simulink model "Demo_Multiple_Quad"  (Simulink 7.7)
settings: Solver=ode4  StartTime=0.0  StopTime=inf  FixedStep=sample_time_Vicon  RelTol=1e-3
InitFcn:
  | sample_time_Vicon = 0.005;
  | sample_time=0.02;
  | DeltaT = sample_time;
  | H0 = 0.35;
  | Kl = 1;
  | Omega_r =1.2; %1.3
  | omega_circle = 36*pi/180;
  | PI = pi;
undefined symbols (not defined in the file or in its folder): DiscIntNeverNeededParam
libraries: simulink x22, dspadpt3 x8
(part 2 of 4)

== system Demo_Multiple_Quad/Quad 6 Planning/Yaw Controller ==
  UAV Bus : Inport
  Bus Selector1 : BusSelector  OutputSignals=Attitude,attitude des,rc
  Gain : Gain  Gain=180/pi
  Heading : simulink/Continuous/PID Controller  SystemSampleTime=-1  Controller=PI  TimeDomain=Discrete-time  SampleTime=sample_time  IntegratorMethod=Trapezoidal  FilterMethod=Trapezoidal  Form=Parallel  P=2  I=1  D=0  N=100  InitialConditionSource=internal  InitialConditionForIntegrator=0  InitialConditionForFilter=0  ExternalReset=rising  LimitOutput=on  UpperSaturationLimit=300*pi/180  LowerSaturationLimit=-300*pi/180  LinearizeAsGain=off  AntiWindupMode=none  Kb=1  TrackingMode=off  Kt=1  PParamMin=[]  PParamMax=[]  IParamMin=[]  IParamMax=[]  DParamMin=[]  DParamMax=[]  NParamMin=[]  NParamMax=[]  KbParamMin=[]  KbParamMax=[]  KtParamMin=[]  KtParamMax=[]  POutMin=[]  POutMax=[]  IOutMin=[]  IOutMax=[]  DOutMin=[]  DOutMax=[]  NOutMin=[]  NOutMax=[]  KbOutMin=[]  KbOutMax=[]  KtOutMin=[]  KtOutMax=[]  IntegratorOutMin=[]  IntegratorOutMax=[]  FilterOutMin=[]  FilterOutMax=[]  SumOutMin=[]  SumOutMax=[]  SumI1OutMin=[]  SumI1OutMax=[]  SumI2OutMin=[]  SumI2OutMax=[]  SumI3OutMin=[]  SumI3OutMax=[]  SumDOutMin=[]  SumDOutMax=[]  SaturationOutMin=[]  SaturationOutMax=[]  IntegratorContinuousStateAttributes=''  IntegratorStateMustResolveToSignalObject=off  IntegratorRTWStateStorageClass=Auto  FilterContinuousStateAttributes=''  FilterStateMustResolveToSignalObject=off  FilterRTWStateStorageClass=Auto
  MATLAB Function : Stateflow chart  TreatAsAtomicUnit=on
  Selector5 : Selector  InputPortWidth=3  IndexOptions=Index vector (dialog)  Indices=[3]  OutputSizes=1
  Selector6 : Selector  InputPortWidth=3  IndexOptions=Index vector (dialog)  Indices=[3]  OutputSizes=1
  Selector7 : Selector  InputPortWidth=8  IndexOptions=Index vector (dialog)  Indices=[5]  OutputSizes=1
  Sum1 : Sum  Inputs=|-+
  Yaw rate des : Outport
  wires:
  Bus Selector1/3 -> Selector7/1  "<rc>"
  Bus Selector1/2 -> Selector6/1  "<attitude des>"
  Selector6/1 -> Sum1/2
  Sum1/1 -> MATLAB Function/1(u)
  MATLAB Function/1(y) -> Heading/1
  UAV Bus/1 -> Bus Selector1/1
  Bus Selector1/1 -> Selector5/1  "<Attitude>"
  Heading/1 -> Gain/1  "desire yaw rate"
  Selector7/1 -> Heading/2  "reset"
  Selector5/1 -> Sum1/1
  Gain/1 -> Yaw rate des/1

== system Demo_Multiple_Quad/Quad 7 Planning/Horizontal Pos controller ==
  UAV Bus : Inport
  Bus Selector : BusSelector  OutputSignals=Position,position des
  Horizontal Position Controller : Subsystem
  Mux : Mux  Inputs=2
  p vs pdes : Scope
      settings: YMin=-1.1  YMax=0.5
  RPY : Outport
  wires:
  UAV Bus/1 -> Horizontal Position Controller/1(UAV Bus), Bus Selector/1
  Horizontal Position Controller/1(RPY) -> RPY/1
  Bus Selector/1 -> Mux/1  "<Position>"
  Bus Selector/2 -> Mux/2  "<position des>"
  Mux/1 -> p vs pdes/1

== system Demo_Multiple_Quad/Quad 7 Planning/Mixer ==
  note: 7x1 vector (usec, XYZRPY)
  RP : Inport
  T : Inport  Port=2
  Yaw rate : Inport  Port=3
  Gain : Gain  Gain=180/pi
  Mux1 : Mux  Inputs=5
  PWM : Constant  Value=0
  "[-1, 1]" : Fcn  Expr=u(1)*2-1
  id : Constant  Value=7
  XYZ RPY : Outport
  wires:
  Mux1/1 -> XYZ RPY/1
  T/1 -> "[-1, 1]"/1
  RP/1 -> Gain/1
  Yaw rate/1 -> Mux1/3
  PWM/1 -> Mux1/4
  id/1 -> Mux1/5
  Gain/1 -> Mux1/2
  "[-1, 1]"/1 -> Mux1/1

== system Demo_Multiple_Quad/Quad 7 Planning/Trajectory Logic ==
  UAV Bus : Inport
  PerchPos : Inport  Port=2
  Bus Selector : BusSelector  OutputSignals=rc,Position,Attitude
  CommandRefSystem : Subsystem
  Mux : Mux  Inputs=2
  Selector1 : Selector  InputPortWidth=3  IndexOptions=Index vector (dialog)  Indices=[3]  OutputSizes=1
  UAV SF1 : Stateflow chart  TreatAsAtomicUnit=on
  PosRef : Outport
  attitude des : Outport  Port=2
  VelRef : Outport  Port=3
  AccRef : Outport  Port=4
  HoverThrottle : Outport  Port=5
  Mode : Outport  Port=6
  wires:
  UAV SF1/1(PosDesired) -> CommandRefSystem/1(PosCom)
  CommandRefSystem/1(position des) -> PosRef/1
  CommandRefSystem/3(velocity des) -> VelRef/1
  Bus Selector/1 -> UAV SF1/1(RC)  "<rc>"
  CommandRefSystem/4(acc des) -> AccRef/1
  UAV SF1/2(HoverThrottle) -> HoverThrottle/1
  PerchPos/1 -> UAV SF1/3(PerchPos)
  UAV SF1/3(Mode) -> Mode/1
  UAV Bus/1 -> Bus Selector/1
  CommandRefSystem/2(attitude des) -> attitude des/1
  Bus Selector/2 -> Mux/1  "<Position>"
  Bus Selector/3 -> Selector1/1  "<Attitude>"
  Selector1/1 -> Mux/2
  Mux/1 -> UAV SF1/2(Pos)

== system Demo_Multiple_Quad/Quad 7 Planning/Vertical Controller ==
  note: Manual Thrust
  UAV bus : Inport
  Hover Throttle : Inport  Port=2
  RP Cmd : Inport  Port=3
  Bus Selector : BusSelector  OutputSignals=Position,position des,rc,velocity,velocity des
  Bus Selector3 : BusSelector  OutputSignals=rc
  Compensation for T from RP cmd : Fcn  Expr=u(1)/(cos(u(2))*cos(u(3)))
  Mux1 : Mux  Inputs=2
  Selector{1,3..5} (4 alike) : Selector  InputPortWidth=3  IndexOptions=Index vector (dialog)  Indices=[3]  OutputSizes=1
  Selector2 : Selector  InputPortWidth=8  IndexOptions=Index vector (dialog)  Indices=[1]  OutputSizes=1
  Selector7 : Selector  InputPortWidth=8  IndexOptions=Index vector (dialog)  Indices=[7]  OutputSizes=1
  Sum : Sum  Inputs=|-+
  Sum1 : Sum  Inputs=|-+
  Verticall Pos Controller : Subsystem
  T : Outport
  wires:
  UAV bus/1 -> Bus Selector/1
  Bus Selector/3 -> Bus Selector3/1, Selector2/1  "<rc>"
  Bus Selector/1 -> Selector4/1  "<Position>"
  Bus Selector/2 -> Selector1/1  "<position des>"
  Sum/1 -> Verticall Pos Controller/1(Pos Error)  "Down error"
  Selector4/1 -> Sum/1
  Selector1/1 -> Sum/2
  Bus Selector3/1 -> Selector7/1  "<rc>"
  Selector7/1 -> Verticall Pos Controller/2(Reset)  "reset"
  Sum1/1 -> Verticall Pos Controller/3(Vel Error)  "Vel_error"
  Selector3/1 -> Sum1/1
  Selector5/1 -> Sum1/2
  Bus Selector/4 -> Selector3/1  "<velocity>"
  Bus Selector/5 -> Selector5/1  "<velocity des>"
  Hover Throttle/1 -> Verticall Pos Controller/4(Hover Throttle)
  RP Cmd/1 -> Mux1/2
  Mux1/1 -> Compensation for T from RP cmd/1
  Verticall Pos Controller/1("T  Commands [0, 1]") -> Mux1/1  "T"
  Compensation for T from RP cmd/1 -> T/1

== system Demo_Multiple_Quad/Quad 7 Planning/Yaw Controller ==
  UAV Bus : Inport
  Bus Selector1 : BusSelector  OutputSignals=Attitude,attitude des,rc
  Gain : Gain  Gain=180/pi
  Heading : simulink/Continuous/PID Controller  SystemSampleTime=-1  Controller=PI  TimeDomain=Discrete-time  SampleTime=sample_time  IntegratorMethod=Trapezoidal  FilterMethod=Trapezoidal  Form=Parallel  P=2  I=1  D=0  N=100  InitialConditionSource=internal  InitialConditionForIntegrator=0  InitialConditionForFilter=0  ExternalReset=rising  LimitOutput=on  UpperSaturationLimit=300*pi/180  LowerSaturationLimit=-300*pi/180  LinearizeAsGain=off  AntiWindupMode=none  Kb=1  TrackingMode=off  Kt=1  PParamMin=[]  PParamMax=[]  IParamMin=[]  IParamMax=[]  DParamMin=[]  DParamMax=[]  NParamMin=[]  NParamMax=[]  KbParamMin=[]  KbParamMax=[]  KtParamMin=[]  KtParamMax=[]  POutMin=[]  POutMax=[]  IOutMin=[]  IOutMax=[]  DOutMin=[]  DOutMax=[]  NOutMin=[]  NOutMax=[]  KbOutMin=[]  KbOutMax=[]  KtOutMin=[]  KtOutMax=[]  IntegratorOutMin=[]  IntegratorOutMax=[]  FilterOutMin=[]  FilterOutMax=[]  SumOutMin=[]  SumOutMax=[]  SumI1OutMin=[]  SumI1OutMax=[]  SumI2OutMin=[]  SumI2OutMax=[]  SumI3OutMin=[]  SumI3OutMax=[]  SumDOutMin=[]  SumDOutMax=[]  SaturationOutMin=[]  SaturationOutMax=[]  IntegratorContinuousStateAttributes=''  IntegratorStateMustResolveToSignalObject=off  IntegratorRTWStateStorageClass=Auto  FilterContinuousStateAttributes=''  FilterStateMustResolveToSignalObject=off  FilterRTWStateStorageClass=Auto
  MATLAB Function : Stateflow chart  TreatAsAtomicUnit=on
  Selector5 : Selector  InputPortWidth=3  IndexOptions=Index vector (dialog)  Indices=[3]  OutputSizes=1
  Selector6 : Selector  InputPortWidth=3  IndexOptions=Index vector (dialog)  Indices=[3]  OutputSizes=1
  Selector7 : Selector  InputPortWidth=8  IndexOptions=Index vector (dialog)  Indices=[5]  OutputSizes=1
  Sum1 : Sum  Inputs=|-+
  Yaw rate des : Outport
  wires:
  Gain/1 -> Yaw rate des/1
  Selector5/1 -> Sum1/1
  Selector7/1 -> Heading/2  "reset"
  Heading/1 -> Gain/1  "desire yaw rate"
  Bus Selector1/1 -> Selector5/1  "<Attitude>"
  UAV Bus/1 -> Bus Selector1/1
  MATLAB Function/1(y) -> Heading/1
  Sum1/1 -> MATLAB Function/1(u)
  Selector6/1 -> Sum1/2
  Bus Selector1/2 -> Selector6/1  "<attitude des>"
  Bus Selector1/3 -> Selector7/1  "<rc>"

== system Demo_Multiple_Quad/Quad 8 Planning /Horizontal Pos controller ==
  UAV Bus : Inport
  Bus Selector : BusSelector  OutputSignals=Position,Attitude,velocity,position des,attitude des,velocity des,rc,Acc des
  Horizontal Position Controller : Subsystem
  RP Cmd : Outport
  wires:
  Horizontal Position Controller/1(RP Cmd) -> RP Cmd/1
  UAV Bus/1 -> Bus Selector/1, Horizontal Position Controller/1(UAV Bus)

== system Demo_Multiple_Quad/Quad 8 Planning /Mixer ==
  note: 7x1 vector (usec, XYZRPY)
  RP : Inport
  T : Inport  Port=2
  Yaw rate : Inport  Port=3
  Gain : Gain  Gain=180/pi
  Mux1 : Mux  Inputs=5
  PWM : Constant  Value=0
  "[-1, 1]" : Fcn  Expr=u(1)*2-1
  id : Constant  Value=8
  XYZ RPY : Outport
  wires:
  id/1 -> Mux1/5
  PWM/1 -> Mux1/4
  Yaw rate/1 -> Mux1/3
  RP/1 -> Gain/1
  T/1 -> "[-1, 1]"/1
  Mux1/1 -> XYZ RPY/1
  Gain/1 -> Mux1/2
  "[-1, 1]"/1 -> Mux1/1

== system Demo_Multiple_Quad/Quad 8 Planning /Trajectory Logic ==
  UAV Bus : Inport
  PerchPos : Inport  Port=2
  Bus Selector : BusSelector  OutputSignals=rc,Position,Attitude
  CommandRefSystem : Subsystem
  Mux : Mux  Inputs=2
  Selector1 : Selector  InputPortWidth=3  IndexOptions=Index vector (dialog)  Indices=[3]  OutputSizes=1
  UAV SF : Stateflow chart  TreatAsAtomicUnit=on
  PosRef : Outport
  attitude des : Outport  Port=2
  VelRef : Outport  Port=3
  AccRef : Outport  Port=4
  HoverThrottle : Outport  Port=5
  Mode : Outport  Port=6
  wires:
  Mux/1 -> UAV SF/2(Pos)
  Selector1/1 -> Mux/2
  Bus Selector/3 -> Selector1/1  "<Attitude>"
  Bus Selector/2 -> Mux/1  "<Position>"
  CommandRefSystem/2(attitude des) -> attitude des/1
  UAV Bus/1 -> Bus Selector/1
  UAV SF/3(Mode) -> Mode/1
  PerchPos/1 -> UAV SF/3(PerchPos)
  UAV SF/2(HoverThrottle) -> HoverThrottle/1
  CommandRefSystem/4(acc des) -> AccRef/1
  Bus Selector/1 -> UAV SF/1(RC)  "<rc>"
  CommandRefSystem/3(velocity des) -> VelRef/1
  CommandRefSystem/1(position des) -> PosRef/1
  UAV SF/1(PosDesired) -> CommandRefSystem/1(PosCom)

== system Demo_Multiple_Quad/Quad 8 Planning /Vertical Controller ==
  note: Manual Thrust
  UAV bus : Inport
  Hover Throttle : Inport  Port=2
  RP Cmd : Inport  Port=3
  Bus Selector : BusSelector  OutputSignals=Position,position des,rc,velocity,velocity des
  Bus Selector3 : BusSelector  OutputSignals=rc
  Compensation for T from RP cmd : Fcn  Expr=u(1)/(cos(u(2))*cos(u(3)))
  Mux1 : Mux  Inputs=2
  Selector{1,3..5} (4 alike) : Selector  InputPortWidth=3  IndexOptions=Index vector (dialog)  Indices=[3]  OutputSizes=1
  Selector2 : Selector  InputPortWidth=8  IndexOptions=Index vector (dialog)  Indices=[1]  OutputSizes=1
  Selector7 : Selector  InputPortWidth=8  IndexOptions=Index vector (dialog)  Indices=[7]  OutputSizes=1
  Sum : Sum  Inputs=|-+
  Sum1 : Sum  Inputs=|-+
  Verticall Pos Controller : Subsystem
  T : Outport
  wires:
  Compensation for T from RP cmd/1 -> T/1
  Mux1/1 -> Compensation for T from RP cmd/1
  RP Cmd/1 -> Mux1/2
  Hover Throttle/1 -> Verticall Pos Controller/4(Hover Throttle)
  Verticall Pos Controller/1("T  Commands [0, 1]") -> Mux1/1  "T"
  Bus Selector/5 -> Selector5/1  "<velocity des>"
  Bus Selector/4 -> Selector3/1  "<velocity>"
  Selector5/1 -> Sum1/2
  Selector3/1 -> Sum1/1
  Sum1/1 -> Verticall Pos Controller/3(Vel Error)  "Vel_error"
  Selector7/1 -> Verticall Pos Controller/2(Reset)  "reset"
  Bus Selector3/1 -> Selector7/1  "<rc>"
  Selector1/1 -> Sum/2
  Selector4/1 -> Sum/1
  Sum/1 -> Verticall Pos Controller/1(Pos Error)  "Down error"
  Bus Selector/2 -> Selector1/1  "<position des>"
  Bus Selector/1 -> Selector4/1  "<Position>"
  Bus Selector/3 -> Selector2/1, Bus Selector3/1  "<rc>"
  UAV bus/1 -> Bus Selector/1

== system Demo_Multiple_Quad/Quad 8 Planning /Yaw Controller ==
  UAV Bus : Inport
  Bus Selector1 : BusSelector  OutputSignals=Attitude,attitude des,rc
  Gain : Gain  Gain=180/pi
  Heading : simulink/Continuous/PID Controller  SystemSampleTime=-1  Controller=PI  TimeDomain=Discrete-time  SampleTime=sample_time  IntegratorMethod=Trapezoidal  FilterMethod=Trapezoidal  Form=Parallel  P=2  I=1  D=0  N=100  InitialConditionSource=internal  InitialConditionForIntegrator=0  InitialConditionForFilter=0  ExternalReset=rising  LimitOutput=on  UpperSaturationLimit=300*pi/180  LowerSaturationLimit=-300*pi/180  LinearizeAsGain=off  AntiWindupMode=none  Kb=1  TrackingMode=off  Kt=1  PParamMin=[]  PParamMax=[]  IParamMin=[]  IParamMax=[]  DParamMin=[]  DParamMax=[]  NParamMin=[]  NParamMax=[]  KbParamMin=[]  KbParamMax=[]  KtParamMin=[]  KtParamMax=[]  POutMin=[]  POutMax=[]  IOutMin=[]  IOutMax=[]  DOutMin=[]  DOutMax=[]  NOutMin=[]  NOutMax=[]  KbOutMin=[]  KbOutMax=[]  KtOutMin=[]  KtOutMax=[]  IntegratorOutMin=[]  IntegratorOutMax=[]  FilterOutMin=[]  FilterOutMax=[]  SumOutMin=[]  SumOutMax=[]  SumI1OutMin=[]  SumI1OutMax=[]  SumI2OutMin=[]  SumI2OutMax=[]  SumI3OutMin=[]  SumI3OutMax=[]  SumDOutMin=[]  SumDOutMax=[]  SaturationOutMin=[]  SaturationOutMax=[]  IntegratorContinuousStateAttributes=''  IntegratorStateMustResolveToSignalObject=off  IntegratorRTWStateStorageClass=Auto  FilterContinuousStateAttributes=''  FilterStateMustResolveToSignalObject=off  FilterRTWStateStorageClass=Auto
  MATLAB Function : Stateflow chart  TreatAsAtomicUnit=on
  Selector5 : Selector  InputPortWidth=3  IndexOptions=Index vector (dialog)  Indices=[3]  OutputSizes=1
  Selector6 : Selector  InputPortWidth=3  IndexOptions=Index vector (dialog)  Indices=[3]  OutputSizes=1
  Selector7 : Selector  InputPortWidth=8  IndexOptions=Index vector (dialog)  Indices=[5]  OutputSizes=1
  Sum1 : Sum  Inputs=|-+
  Yaw rate des : Outport
  wires:
  Bus Selector1/3 -> Selector7/1  "<rc>"
  Bus Selector1/2 -> Selector6/1  "<attitude des>"
  Selector6/1 -> Sum1/2
  Sum1/1 -> MATLAB Function/1(u)
  MATLAB Function/1(y) -> Heading/1
  UAV Bus/1 -> Bus Selector1/1
  Bus Selector1/1 -> Selector5/1  "<Attitude>"
  Heading/1 -> Gain/1  "desire yaw rate"
  Selector7/1 -> Heading/2  "reset"
  Selector5/1 -> Sum1/1
  Gain/1 -> Yaw rate des/1

== system Demo_Multiple_Quad/Vicon_Data/Filter1 ==
  In1 : Inport
  Gain : Gain  Gain=15
  Integrator : Integrator
  Kalman Filter : dspadpt3/Kalman Filter  SystemSampleTime=-1  num_targets=1  sourceEnable=Always  isReset=on  X=zeros([9, 1])  P=zeros(9)  A=[1 sample_time_Vicon sample_time_Vicon*sample_time_Vicon/2 zeros(1,6);0 1 sample_time_Vicon zeros(1,6);0 0 1 zeros(1,6);0 0 0 1 sample_time_Vicon sample_time_Vicon*sample_time_Vicon/2 0 0 0;zeros(1,4) 1 sample_time_Vicon zeros(1,3);zeros(1,5) 1 zeros(1,3);zeros(1,6) 1 sample_time_Vicon sample_time_Vicon*sample_time_Vicon/2;zeros(1,7) 1 sample_time_Vicon;zeros(1,8) 1]  sourceMeasure=Specify via Dialog  H=[1 zeros(1,8); zeros(1,3) 1 zeros(1,5);zeros(1,6) 1 0 0]  Q=diag([0 0.001 0.001 0 0.001 0.001 0 0.001 0.001])  R=0.001*eye(3)  isOutputEstMeasure=on  isOutputEstState=on  isOutputEstError=off  isOutputPrdMeasure=off  isOutputPrdState=off  isOutputPrdError=off
  Selector5 : Selector  InputPortWidth=9  IndexOptions=Index vector (dialog)  Indices=[2 5 8]  OutputSizes=1
  Selector6 : Selector  InputPortWidth=9  IndexOptions=Index vector (dialog)  Indices=[3 6 9]  OutputSizes=1
  Sum : Sum  Inputs=|+-
  Pos : Outport
  Vel : Outport  Port=2
  Acc : Outport  Port=3
  wires:
  Selector5/1 -> Vel/1
  Sum/1 -> Gain/1
  Gain/1 -> Integrator/1
  Integrator/1 -> Pos/1, Sum/2
  In1/1 -> Kalman Filter/1, Sum/1
  Kalman Filter/2 -> Selector5/1, Selector6/1
  Selector6/1 -> Acc/1

== system Demo_Multiple_Quad/Vicon_Data/Filter2 ==
  In1 : Inport
  Gain : Gain  Gain=15
  Integrator : Integrator
  Kalman Filter : dspadpt3/Kalman Filter  SystemSampleTime=-1  num_targets=1  sourceEnable=Always  isReset=on  X=zeros([9, 1])  P=zeros(9)  A=[1 sample_time_Vicon sample_time_Vicon*sample_time_Vicon/2 zeros(1,6);0 1 sample_time_Vicon zeros(1,6);0 0 1 zeros(1,6);0 0 0 1 sample_time_Vicon sample_time_Vicon*sample_time_Vicon/2 0 0 0;zeros(1,4) 1 sample_time_Vicon zeros(1,3);zeros(1,5) 1 zeros(1,3);zeros(1,6) 1 sample_time_Vicon sample_time_Vicon*sample_time_Vicon/2;zeros(1,7) 1 sample_time_Vicon;zeros(1,8) 1]  sourceMeasure=Specify via Dialog  H=[1 zeros(1,8); zeros(1,3) 1 zeros(1,5);zeros(1,6) 1 0 0]  Q=diag([0 0.001 0.001 0 0.001 0.001 0 0.001 0.001])  R=0.001*eye(3)  isOutputEstMeasure=on  isOutputEstState=on  isOutputEstError=off  isOutputPrdMeasure=off  isOutputPrdState=off  isOutputPrdError=off
  Selector5 : Selector  InputPortWidth=9  IndexOptions=Index vector (dialog)  Indices=[2 5 8]  OutputSizes=1
  Selector6 : Selector  InputPortWidth=9  IndexOptions=Index vector (dialog)  Indices=[3 6 9]  OutputSizes=1
  Sum : Sum  Inputs=|+-
  Pos : Outport
  Vel : Outport  Port=2
  Acc : Outport  Port=3
  wires:
  Selector6/1 -> Acc/1
  Kalman Filter/2 -> Selector6/1, Selector5/1
  In1/1 -> Sum/1, Kalman Filter/1
  Integrator/1 -> Sum/2, Pos/1
  Gain/1 -> Integrator/1
  Sum/1 -> Gain/1
  Selector5/1 -> Vel/1

== system Demo_Multiple_Quad/Vicon_Data/Filter3 ==
  In1 : Inport
  Gain : Gain  Gain=15
  Integrator : Integrator
  Kalman Filter : dspadpt3/Kalman Filter  SystemSampleTime=-1  num_targets=1  sourceEnable=Always  isReset=on  X=zeros([9, 1])  P=zeros(9)  A=[1 sample_time_Vicon sample_time_Vicon*sample_time_Vicon/2 zeros(1,6);0 1 sample_time_Vicon zeros(1,6);0 0 1 zeros(1,6);0 0 0 1 sample_time_Vicon sample_time_Vicon*sample_time_Vicon/2 0 0 0;zeros(1,4) 1 sample_time_Vicon zeros(1,3);zeros(1,5) 1 zeros(1,3);zeros(1,6) 1 sample_time_Vicon sample_time_Vicon*sample_time_Vicon/2;zeros(1,7) 1 sample_time_Vicon;zeros(1,8) 1]  sourceMeasure=Specify via Dialog  H=[1 zeros(1,8); zeros(1,3) 1 zeros(1,5);zeros(1,6) 1 0 0]  Q=diag([0 0.001 0.001 0 0.001 0.001 0 0.001 0.001])  R=0.001*eye(3)  isOutputEstMeasure=on  isOutputEstState=on  isOutputEstError=off  isOutputPrdMeasure=off  isOutputPrdState=off  isOutputPrdError=off
  Selector5 : Selector  InputPortWidth=9  IndexOptions=Index vector (dialog)  Indices=[2 5 8]  OutputSizes=1
  Selector6 : Selector  InputPortWidth=9  IndexOptions=Index vector (dialog)  Indices=[3 6 9]  OutputSizes=1
  Sum : Sum  Inputs=|+-
  Pos : Outport
  Vel : Outport  Port=2
  Acc : Outport  Port=3
  wires:
  Selector5/1 -> Vel/1
  Sum/1 -> Gain/1
  Gain/1 -> Integrator/1
  Integrator/1 -> Pos/1, Sum/2
  In1/1 -> Kalman Filter/1, Sum/1
  Kalman Filter/2 -> Selector5/1, Selector6/1
  Selector6/1 -> Acc/1

== system Demo_Multiple_Quad/Vicon_Data/Filter4 ==
  In1 : Inport
  Gain : Gain  Gain=15
  Integrator : Integrator
  Kalman Filter : dspadpt3/Kalman Filter  SystemSampleTime=-1  num_targets=1  sourceEnable=Always  isReset=on  X=zeros([9, 1])  P=zeros(9)  A=[1 sample_time_Vicon sample_time_Vicon*sample_time_Vicon/2 zeros(1,6);0 1 sample_time_Vicon zeros(1,6);0 0 1 zeros(1,6);0 0 0 1 sample_time_Vicon sample_time_Vicon*sample_time_Vicon/2 0 0 0;zeros(1,4) 1 sample_time_Vicon zeros(1,3);zeros(1,5) 1 zeros(1,3);zeros(1,6) 1 sample_time_Vicon sample_time_Vicon*sample_time_Vicon/2;zeros(1,7) 1 sample_time_Vicon;zeros(1,8) 1]  sourceMeasure=Specify via Dialog  H=[1 zeros(1,8); zeros(1,3) 1 zeros(1,5);zeros(1,6) 1 0 0]  Q=diag([0 0.001 0.001 0 0.001 0.001 0 0.001 0.001])  R=0.001*eye(3)  isOutputEstMeasure=on  isOutputEstState=on  isOutputEstError=off  isOutputPrdMeasure=off  isOutputPrdState=off  isOutputPrdError=off
  Selector5 : Selector  InputPortWidth=9  IndexOptions=Index vector (dialog)  Indices=[2 5 8]  OutputSizes=1
  Selector6 : Selector  InputPortWidth=9  IndexOptions=Index vector (dialog)  Indices=[3 6 9]  OutputSizes=1
  Sum : Sum  Inputs=|+-
  Pos : Outport
  Vel : Outport  Port=2
  Acc : Outport  Port=3
  wires:
  Selector6/1 -> Acc/1
  Kalman Filter/2 -> Selector6/1, Selector5/1
  In1/1 -> Sum/1, Kalman Filter/1
  Integrator/1 -> Sum/2, Pos/1
  Gain/1 -> Integrator/1
  Sum/1 -> Gain/1
  Selector5/1 -> Vel/1

== system Demo_Multiple_Quad/Vicon_Data/Filter5 ==
  In1 : Inport
  Gain : Gain  Gain=15
  Integrator : Integrator
  Kalman Filter : dspadpt3/Kalman Filter  SystemSampleTime=-1  num_targets=1  sourceEnable=Always  isReset=on  X=zeros([9, 1])  P=zeros(9)  A=[1 sample_time_Vicon sample_time_Vicon*sample_time_Vicon/2 zeros(1,6);0 1 sample_time_Vicon zeros(1,6);0 0 1 zeros(1,6);0 0 0 1 sample_time_Vicon sample_time_Vicon*sample_time_Vicon/2 0 0 0;zeros(1,4) 1 sample_time_Vicon zeros(1,3);zeros(1,5) 1 zeros(1,3);zeros(1,6) 1 sample_time_Vicon sample_time_Vicon*sample_time_Vicon/2;zeros(1,7) 1 sample_time_Vicon;zeros(1,8) 1]  sourceMeasure=Specify via Dialog  H=[1 zeros(1,8); zeros(1,3) 1 zeros(1,5);zeros(1,6) 1 0 0]  Q=diag([0 0.001 0.001 0 0.001 0.001 0 0.001 0.001])  R=0.001*eye(3)  isOutputEstMeasure=on  isOutputEstState=on  isOutputEstError=off  isOutputPrdMeasure=off  isOutputPrdState=off  isOutputPrdError=off
  Selector5 : Selector  InputPortWidth=9  IndexOptions=Index vector (dialog)  Indices=[2 5 8]  OutputSizes=1
  Selector6 : Selector  InputPortWidth=9  IndexOptions=Index vector (dialog)  Indices=[3 6 9]  OutputSizes=1
  Sum : Sum  Inputs=|+-
  Pos : Outport
  Vel : Outport  Port=2
  Acc : Outport  Port=3
  wires:
  Selector5/1 -> Vel/1
  Sum/1 -> Gain/1
  Gain/1 -> Integrator/1
  Integrator/1 -> Pos/1, Sum/2
  In1/1 -> Kalman Filter/1, Sum/1
  Kalman Filter/2 -> Selector5/1, Selector6/1
  Selector6/1 -> Acc/1

== system Demo_Multiple_Quad/Vicon_Data/Filter6 ==
  In1 : Inport
  Gain : Gain  Gain=15
  Integrator : Integrator
  Kalman Filter : dspadpt3/Kalman Filter  SystemSampleTime=-1  num_targets=1  sourceEnable=Always  isReset=on  X=zeros([9, 1])  P=zeros(9)  A=[1 sample_time_Vicon sample_time_Vicon*sample_time_Vicon/2 zeros(1,6);0 1 sample_time_Vicon zeros(1,6);0 0 1 zeros(1,6);0 0 0 1 sample_time_Vicon sample_time_Vicon*sample_time_Vicon/2 0 0 0;zeros(1,4) 1 sample_time_Vicon zeros(1,3);zeros(1,5) 1 zeros(1,3);zeros(1,6) 1 sample_time_Vicon sample_time_Vicon*sample_time_Vicon/2;zeros(1,7) 1 sample_time_Vicon;zeros(1,8) 1]  sourceMeasure=Specify via Dialog  H=[1 zeros(1,8); zeros(1,3) 1 zeros(1,5);zeros(1,6) 1 0 0]  Q=diag([0 0.001 0.001 0 0.001 0.001 0 0.001 0.001])  R=0.001*eye(3)  isOutputEstMeasure=on  isOutputEstState=on  isOutputEstError=off  isOutputPrdMeasure=off  isOutputPrdState=off  isOutputPrdError=off
  Selector5 : Selector  InputPortWidth=9  IndexOptions=Index vector (dialog)  Indices=[2 5 8]  OutputSizes=1
  Selector6 : Selector  InputPortWidth=9  IndexOptions=Index vector (dialog)  Indices=[3 6 9]  OutputSizes=1
  Sum : Sum  Inputs=|+-
  Pos : Outport
  Vel : Outport  Port=2
  Acc : Outport  Port=3
  wires:
  Selector6/1 -> Acc/1
  Kalman Filter/2 -> Selector6/1, Selector5/1
  In1/1 -> Sum/1, Kalman Filter/1
  Integrator/1 -> Sum/2, Pos/1
  Gain/1 -> Integrator/1
  Sum/1 -> Gain/1
  Selector5/1 -> Vel/1

== system Demo_Multiple_Quad/Vicon_Data/Filter7 ==
  In1 : Inport
  Gain : Gain  Gain=15
  Integrator : Integrator
  Kalman Filter : dspadpt3/Kalman Filter  SystemSampleTime=-1  num_targets=1  sourceEnable=Always  isReset=on  X=zeros([9, 1])  P=zeros(9)  A=[1 sample_time_Vicon sample_time_Vicon*sample_time_Vicon/2 zeros(1,6);0 1 sample_time_Vicon zeros(1,6);0 0 1 zeros(1,6);0 0 0 1 sample_time_Vicon sample_time_Vicon*sample_time_Vicon/2 0 0 0;zeros(1,4) 1 sample_time_Vicon zeros(1,3);zeros(1,5) 1 zeros(1,3);zeros(1,6) 1 sample_time_Vicon sample_time_Vicon*sample_time_Vicon/2;zeros(1,7) 1 sample_time_Vicon;zeros(1,8) 1]  sourceMeasure=Specify via Dialog  H=[1 zeros(1,8); zeros(1,3) 1 zeros(1,5);zeros(1,6) 1 0 0]  Q=diag([0 0.001 0.001 0 0.001 0.001 0 0.001 0.001])  R=0.001*eye(3)  isOutputEstMeasure=on  isOutputEstState=on  isOutputEstError=off  isOutputPrdMeasure=off  isOutputPrdState=off  isOutputPrdError=off
  Selector5 : Selector  InputPortWidth=9  IndexOptions=Index vector (dialog)  Indices=[2 5 8]  OutputSizes=1
  Selector6 : Selector  InputPortWidth=9  IndexOptions=Index vector (dialog)  Indices=[3 6 9]  OutputSizes=1
  Sum : Sum  Inputs=|+-
  Pos : Outport
  Vel : Outport  Port=2
  Acc : Outport  Port=3
  wires:
  Selector6/1 -> Acc/1
  Kalman Filter/2 -> Selector6/1, Selector5/1
  In1/1 -> Sum/1, Kalman Filter/1
  Integrator/1 -> Sum/2, Pos/1
  Gain/1 -> Integrator/1
  Sum/1 -> Gain/1
  Selector5/1 -> Vel/1

== system Demo_Multiple_Quad/Vicon_Data/Filter8 ==
  In1 : Inport
  Gain : Gain  Gain=15
  Integrator : Integrator
  Kalman Filter : dspadpt3/Kalman Filter  SystemSampleTime=-1  num_targets=1  sourceEnable=Always  isReset=on  X=zeros([9, 1])  P=zeros(9)  A=[1 sample_time_Vicon sample_time_Vicon*sample_time_Vicon/2 zeros(1,6);0 1 sample_time_Vicon zeros(1,6);0 0 1 zeros(1,6);0 0 0 1 sample_time_Vicon sample_time_Vicon*sample_time_Vicon/2 0 0 0;zeros(1,4) 1 sample_time_Vicon zeros(1,3);zeros(1,5) 1 zeros(1,3);zeros(1,6) 1 sample_time_Vicon sample_time_Vicon*sample_time_Vicon/2;zeros(1,7) 1 sample_time_Vicon;zeros(1,8) 1]  sourceMeasure=Specify via Dialog  H=[1 zeros(1,8); zeros(1,3) 1 zeros(1,5);zeros(1,6) 1 0 0]  Q=diag([0 0.001 0.001 0 0.001 0.001 0 0.001 0.001])  R=0.001*eye(3)  isOutputEstMeasure=on  isOutputEstState=on  isOutputEstError=off  isOutputPrdMeasure=off  isOutputPrdState=off  isOutputPrdError=off
  Selector5 : Selector  InputPortWidth=9  IndexOptions=Index vector (dialog)  Indices=[2 5 8]  OutputSizes=1
  Selector6 : Selector  InputPortWidth=9  IndexOptions=Index vector (dialog)  Indices=[3 6 9]  OutputSizes=1
  Sum : Sum  Inputs=|+-
  Pos : Outport
  Vel : Outport  Port=2
  Acc : Outport  Port=3
  wires:
  Selector5/1 -> Vel/1
  Sum/1 -> Gain/1
  Gain/1 -> Integrator/1
  Integrator/1 -> Pos/1, Sum/2
  In1/1 -> Kalman Filter/1, Sum/1
  Kalman Filter/2 -> Selector5/1, Selector6/1
  Selector6/1 -> Acc/1

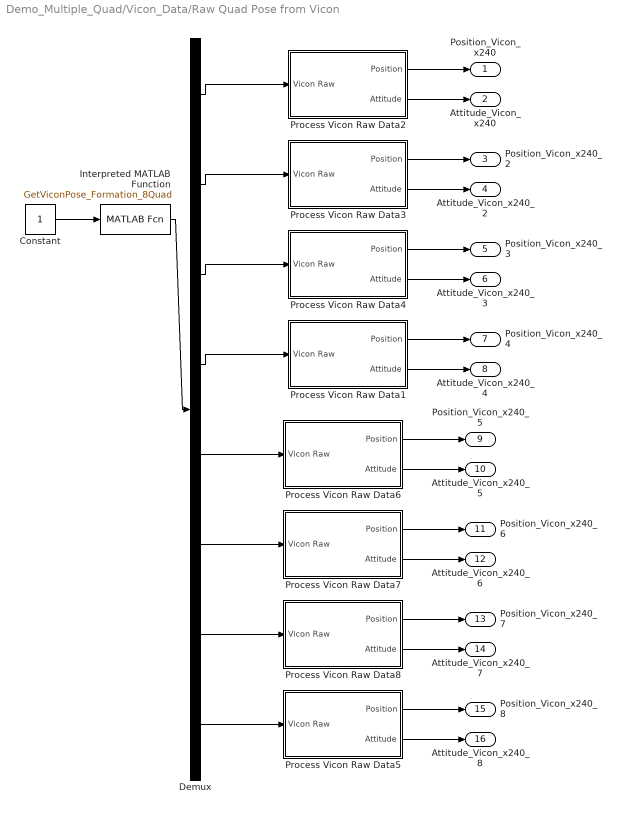
== system Demo_Multiple_Quad/Vicon_Data/Raw Quad Pose from Vicon ==
  Constant : Constant
  Demux : Demux  Outputs=8
  Interpreted MATLAB Function : MATLABFcn  MATLABFcn=GetViconPose_Formation_8Quad
  Process Vicon Raw Data1 : Subsystem
  Process Vicon Raw Data2 : Subsystem
  Process Vicon Raw Data3 : Subsystem
  Process Vicon Raw Data4 : Subsystem
  Process Vicon Raw Data5 : Subsystem
  Process Vicon Raw Data6 : Subsystem
  Process Vicon Raw Data7 : Subsystem
  Process Vicon Raw Data8 : Subsystem
  Position_Vicon_x240 : Outport
  Attitude_Vicon_x240 : Outport  Port=2
  Position_Vicon_x240_2 : Outport  Port=3
  Attitude_Vicon_x240_2 : Outport  Port=4
  Position_Vicon_x240_3 : Outport  Port=5
  Attitude_Vicon_x240_3 : Outport  Port=6
  Position_Vicon_x240_4 : Outport  Port=7
  Attitude_Vicon_x240_4 : Outport  Port=8
  Position_Vicon_x240_5 : Outport  Port=9
  Attitude_Vicon_x240_5 : Outport  Port=10
  Position_Vicon_x240_6 : Outport  Port=11
  Attitude_Vicon_x240_6 : Outport  Port=12
  Position_Vicon_x240_7 : Outport  Port=13
  Attitude_Vicon_x240_7 : Outport  Port=14
  Position_Vicon_x240_8 : Outport  Port=15
  Attitude_Vicon_x240_8 : Outport  Port=16
  wires:
  Process Vicon Raw Data2/2(Attitude) -> Attitude_Vicon_x240/1
  Process Vicon Raw Data2/1(Position) -> Position_Vicon_x240/1
  Constant/1 -> Interpreted MATLAB Function/1
  Interpreted MATLAB Function/1 -> Demux/1
  Process Vicon Raw Data3/2(Attitude) -> Attitude_Vicon_x240_2/1
  Process Vicon Raw Data3/1(Position) -> Position_Vicon_x240_2/1
  Process Vicon Raw Data4/2(Attitude) -> Attitude_Vicon_x240_3/1
  Process Vicon Raw Data4/1(Position) -> Position_Vicon_x240_3/1
  Demux/1 -> Process Vicon Raw Data2/1(Vicon Raw)
  Demux/2 -> Process Vicon Raw Data3/1(Vicon Raw)
  Demux/3 -> Process Vicon Raw Data4/1(Vicon Raw)
  Process Vicon Raw Data1/2(Attitude) -> Attitude_Vicon_x240_4/1
  Process Vicon Raw Data1/1(Position) -> Position_Vicon_x240_4/1
  Demux/4 -> Process Vicon Raw Data1/1(Vicon Raw)
  Process Vicon Raw Data6/2(Attitude) -> Attitude_Vicon_x240_5/1
  Process Vicon Raw Data6/1(Position) -> Position_Vicon_x240_5/1
  Process Vicon Raw Data7/2(Attitude) -> Attitude_Vicon_x240_6/1
  Process Vicon Raw Data7/1(Position) -> Position_Vicon_x240_6/1
  Process Vicon Raw Data8/2(Attitude) -> Attitude_Vicon_x240_7/1
  Process Vicon Raw Data8/1(Position) -> Position_Vicon_x240_7/1
  Demux/5 -> Process Vicon Raw Data6/1(Vicon Raw)
  Demux/6 -> Process Vicon Raw Data7/1(Vicon Raw)
  Demux/7 -> Process Vicon Raw Data8/1(Vicon Raw)
  Process Vicon Raw Data5/2(Attitude) -> Attitude_Vicon_x240_8/1
  Process Vicon Raw Data5/1(Position) -> Position_Vicon_x240_8/1
  Demux/8 -> Process Vicon Raw Data5/1(Vicon Raw)

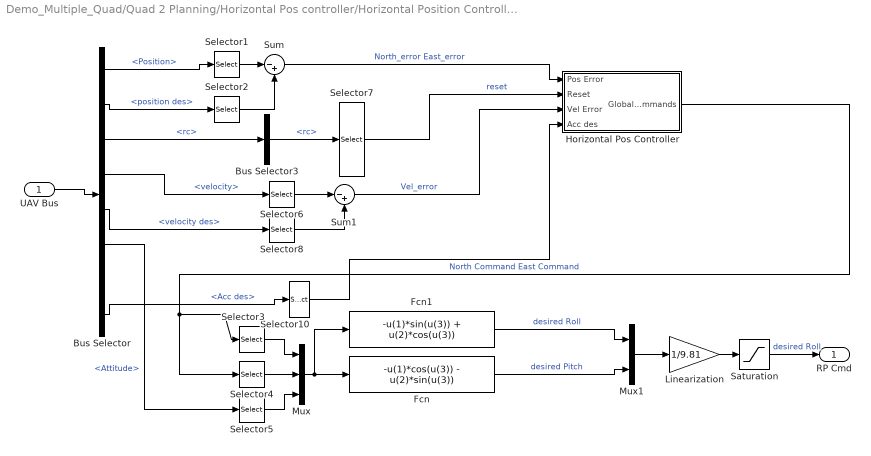
== system Demo_Multiple_Quad/Quad 2 Planning/Horizontal Pos controller/Horizontal Position Controller ==
  UAV Bus : Inport
  Bus Selector : BusSelector  OutputSignals=Position,position des,rc,velocity,velocity des,Attitude,Acceleration,Acc des
  Bus Selector3 : BusSelector  OutputSignals=rc
  Fcn : Fcn  Expr=-u(1)*cos(u(3)) - u(2)*sin(u(3))
  Fcn1 : Fcn  Expr=-u(1)*sin(u(3)) + u(2)*cos(u(3))
  Horizontal Pos Controller : Subsystem
  Linearization : Gain  Gain=1/9.81  OutDataTypeStr=double
  Mux : Mux  Inputs=3
  Mux1 : Mux  Inputs=2
  Saturation : Saturate  UpperLimit=60*pi/180  LowerLimit=-60*pi/180
  Selector{1..2,6,8} (4 alike) : Selector  InputPortWidth=3  IndexOptions=Index vector (dialog)  Indices=[1 2]  OutputSizes=1
  Selector10 : Selector  InputPortWidth=4  IndexOptions=Index vector (dialog)  Indices=[1 2]  OutputSizes=1
  Selector3 : Selector  InputPortWidth=2  IndexOptions=Index vector (dialog)  Indices=[1]  OutputSizes=1
  Selector4 : Selector  InputPortWidth=2  IndexOptions=Index vector (dialog)  Indices=[2]  OutputSizes=1
  Selector5 : Selector  InputPortWidth=3  IndexOptions=Index vector (dialog)  Indices=[3]  OutputSizes=1
  Selector7 : Selector  InputPortWidth=8  IndexOptions=Index vector (dialog)  Indices=[7]  OutputSizes=1
  Sum : Sum  Inputs=|-+
  Sum1 : Sum  Inputs=|-+
  RP Cmd : Outport
  wires:
  Sum/1 -> Horizontal Pos Controller/1(Pos Error)  "North_error East_error"
  Bus Selector/1 -> Selector1/1  "<Position>"
  Bus Selector/2 -> Selector2/1  "<position des>"
  Selector1/1 -> Sum/1
  Selector2/1 -> Sum/2
  UAV Bus/1 -> Bus Selector/1
  Horizontal Pos Controller/1(Global Commands) -> Selector3/1, Selector4/1  "North Command East Command"
  Bus Selector/6 -> Selector5/1  "<Attitude>"
  Selector3/1 -> Mux/1
  Selector4/1 -> Mux/2
  Selector5/1 -> Mux/3
  Mux/1 -> Fcn/1, Fcn1/1
  Fcn1/1 -> Mux1/1  "desired Roll"
  Fcn/1 -> Mux1/2  "desired Pitch"
  Mux1/1 -> Linearization/1
  Bus Selector3/1 -> Selector7/1  "<rc>"
  Selector7/1 -> Horizontal Pos Controller/2(Reset)  "reset"
  Sum1/1 -> Horizontal Pos Controller/3(Vel Error)  "Vel_error"
  Selector6/1 -> Sum1/1
  Selector8/1 -> Sum1/2
  Bus Selector/3 -> Bus Selector3/1  "<rc>"
  Bus Selector/4 -> Selector6/1  "<velocity>"
  Bus Selector/5 -> Selector8/1  "<velocity des>"
  Bus Selector/8 -> Selector10/1  "<Acc des>"
  Selector10/1 -> Horizontal Pos Controller/4(Acc des)
  Linearization/1 -> Saturation/1
  Saturation/1 -> RP Cmd/1  "desired Roll"

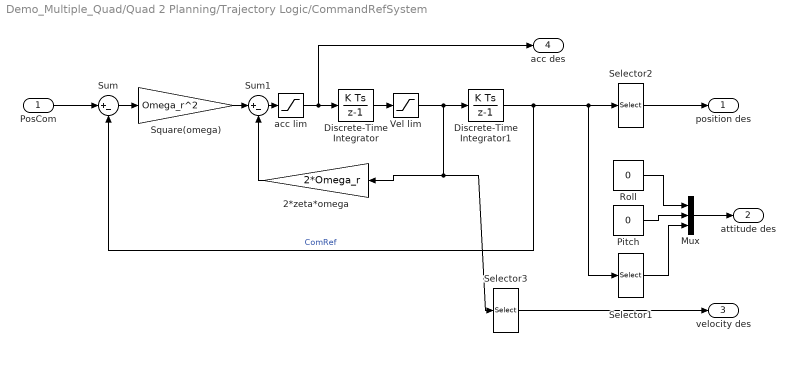
== system Demo_Multiple_Quad/Quad 2 Planning/Trajectory Logic/CommandRefSystem ==
  PosCom : Inport
  2*zeta*omega : Gain  Gain=2*Omega_r
  Discrete-Time Integrator : DiscreteIntegrator  SampleTime=0.02  ICPrevOutput=DiscIntNeverNeededParam  ICPrevScaledInput=DiscIntNeverNeededParam
  Discrete-Time Integrator1 : DiscreteIntegrator  SampleTime=0.02  ICPrevOutput=DiscIntNeverNeededParam  ICPrevScaledInput=DiscIntNeverNeededParam
  Mux : Mux  Inputs=3
  Pitch : Constant  Value=0  SampleTime=0.02
  Roll : Constant  Value=0  SampleTime=0.02
  Selector1 : Selector  InputPortWidth=4  IndexOptions=Index vector (dialog)  Indices=[4]  OutputSizes=1
  Selector2 : Selector  InputPortWidth=4  IndexOptions=Index vector (dialog)  Indices=[1 2 3]  OutputSizes=1
  Selector3 : Selector  InputPortWidth=4  IndexOptions=Index vector (dialog)  Indices=[1 2 3]  OutputSizes=1
  Square(omega) : Gain  Gain=Omega_r^2
  Sum : Sum  Inputs=|+-
  Sum1 : Sum  Inputs=|+-
  Vel lim : Saturate  UpperLimit=3  LowerLimit=-3
  acc lim : Saturate  UpperLimit=4  LowerLimit=-4
  position des : Outport
  attitude des : Outport  Port=2
  velocity des : Outport  Port=3
  acc des : Outport  Port=4
  wires:
  Discrete-Time Integrator1/1 -> Sum/2, Selector2/1, Selector1/1  "ComRef"
  PosCom/1 -> Sum/1
  Sum/1 -> Square(omega)/1
  Square(omega)/1 -> Sum1/1
  Discrete-Time Integrator/1 -> Vel lim/1
  Sum1/1 -> acc lim/1
  2*zeta*omega/1 -> Sum1/2
  Selector2/1 -> position des/1
  Roll/1 -> Mux/1
  Pitch/1 -> Mux/2
  Selector1/1 -> Mux/3
  Mux/1 -> attitude des/1
  Selector3/1 -> velocity des/1
  acc lim/1 -> acc des/1, Discrete-Time Integrator/1
  Vel lim/1 -> 2*zeta*omega/1, Selector3/1, Discrete-Time Integrator1/1

== system Demo_Multiple_Quad/Quad 2 Planning/Vertical Controller/Verticall Pos Controller ==
  note: Set 1:
      | without KF
  note: 0.25
      | 0.1
      | 0.15
  note: Set 1:
      | with KF
  note: 0.15
      | 0.08
      | 0.15
  Pos Error : Inport
  Reset : Inport  Port=2
  Vel Error : Inport  Port=3
  Hover Throttle : Inport  Port=4
  D Gain : Gain  Gain=0.1  OutDataTypeStr=double
  Integral Gain : Gain  DisableCoverage=on  Gain=0.05  ParamDataTypeStr=double  OutDataTypeStr=double
  Integrator : DiscreteIntegrator  DisableCoverage=on  IntegratorMethod=Integration: Trapezoidal  ExternalReset=rising  InitialConditionMode=State only (most efficient)  SampleTime=-1  OutDataTypeStr=double  LimitOutput=on  UpperSaturationLimit=0.3  LowerSaturationLimit=-0.3  ICPrevOutput=DiscIntNeverNeededParam  ICPrevScaledInput=DiscIntNeverNeededParam
  Proportional Gain : Gain  DisableCoverage=on  Gain=0.1  ParamDataTypeStr=double  OutDataTypeStr=double
  Sum1 : Sum  DisableCoverage=on  Inputs=---|  AccumDataTypeStr=double  OutDataTypeStr=double  SampleTime=0.02
  Sum2 : Sum  DisableCoverage=on  Inputs=++|  AccumDataTypeStr=double  OutDataTypeStr=double  SampleTime=0.02
  "T  Commands [0, 1]" : Outport
  wires:
  Integral Gain/1 -> Integrator/1
  Integrator/1 -> Sum1/2
  Proportional Gain/1 -> Sum1/1
  Pos Error/1 -> Proportional Gain/1, Integral Gain/1
  Reset/1 -> Integrator/2
  Vel Error/1 -> D Gain/1
  D Gain/1 -> Sum1/3
  Sum1/1 -> Sum2/1
  Hover Throttle/1 -> Sum2/2
  Sum2/1 -> "T  Commands [0, 1]"/1

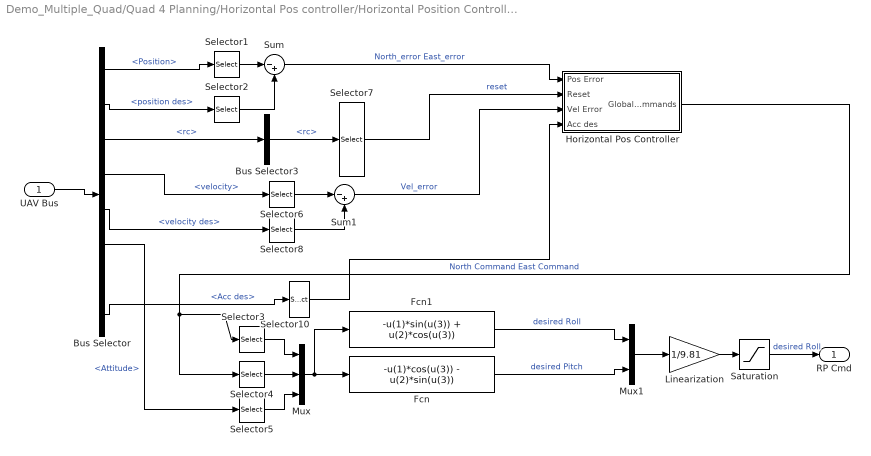
== system Demo_Multiple_Quad/Quad 4 Planning/Horizontal Pos controller/Horizontal Position Controller ==
  UAV Bus : Inport
  Bus Selector : BusSelector  OutputSignals=Position,position des,rc,velocity,velocity des,Attitude,Acceleration,Acc des
  Bus Selector3 : BusSelector  OutputSignals=rc
  Fcn : Fcn  Expr=-u(1)*cos(u(3)) - u(2)*sin(u(3))
  Fcn1 : Fcn  Expr=-u(1)*sin(u(3)) + u(2)*cos(u(3))
  Horizontal Pos Controller : Subsystem
  Linearization : Gain  Gain=1/9.81  OutDataTypeStr=double
  Mux : Mux  Inputs=3
  Mux1 : Mux  Inputs=2
  Saturation : Saturate  UpperLimit=60*pi/180  LowerLimit=-60*pi/180
  Selector{1..2,6,8} (4 alike) : Selector  InputPortWidth=3  IndexOptions=Index vector (dialog)  Indices=[1 2]  OutputSizes=1
  Selector10 : Selector  InputPortWidth=4  IndexOptions=Index vector (dialog)  Indices=[1 2]  OutputSizes=1
  Selector3 : Selector  InputPortWidth=2  IndexOptions=Index vector (dialog)  Indices=[1]  OutputSizes=1
  Selector4 : Selector  InputPortWidth=2  IndexOptions=Index vector (dialog)  Indices=[2]  OutputSizes=1
  Selector5 : Selector  InputPortWidth=3  IndexOptions=Index vector (dialog)  Indices=[3]  OutputSizes=1
  Selector7 : Selector  InputPortWidth=8  IndexOptions=Index vector (dialog)  Indices=[7]  OutputSizes=1
  Sum : Sum  Inputs=|-+
  Sum1 : Sum  Inputs=|-+
  RP Cmd : Outport
  wires:
  Saturation/1 -> RP Cmd/1  "desired Roll"
  Linearization/1 -> Saturation/1
  Selector10/1 -> Horizontal Pos Controller/4(Acc des)
  Bus Selector/8 -> Selector10/1  "<Acc des>"
  Bus Selector/5 -> Selector8/1  "<velocity des>"
  Bus Selector/4 -> Selector6/1  "<velocity>"
  Bus Selector/3 -> Bus Selector3/1  "<rc>"
  Selector8/1 -> Sum1/2
  Selector6/1 -> Sum1/1
  Sum1/1 -> Horizontal Pos Controller/3(Vel Error)  "Vel_error"
  Selector7/1 -> Horizontal Pos Controller/2(Reset)  "reset"
  Bus Selector3/1 -> Selector7/1  "<rc>"
  Mux1/1 -> Linearization/1
  Fcn/1 -> Mux1/2  "desired Pitch"
  Fcn1/1 -> Mux1/1  "desired Roll"
  Mux/1 -> Fcn1/1, Fcn/1
  Selector5/1 -> Mux/3
  Selector4/1 -> Mux/2
  Selector3/1 -> Mux/1
  Bus Selector/6 -> Selector5/1  "<Attitude>"
  Horizontal Pos Controller/1(Global Commands) -> Selector4/1, Selector3/1  "North Command East Command"
  UAV Bus/1 -> Bus Selector/1
  Selector2/1 -> Sum/2
  Selector1/1 -> Sum/1
  Bus Selector/2 -> Selector2/1  "<position des>"
  Bus Selector/1 -> Selector1/1  "<Position>"
  Sum/1 -> Horizontal Pos Controller/1(Pos Error)  "North_error East_error"

== system Demo_Multiple_Quad/Quad 4 Planning/Trajectory Logic/CommandRefSystem ==
  PosCom : Inport
  2*zeta*omega : Gain  Gain=2*Omega_r
  Discrete-Time Integrator : DiscreteIntegrator  SampleTime=0.02  ICPrevOutput=DiscIntNeverNeededParam  ICPrevScaledInput=DiscIntNeverNeededParam
  Discrete-Time Integrator1 : DiscreteIntegrator  SampleTime=0.02  ICPrevOutput=DiscIntNeverNeededParam  ICPrevScaledInput=DiscIntNeverNeededParam
  Mux : Mux  Inputs=3
  Pitch : Constant  Value=0  SampleTime=0.02
  Roll : Constant  Value=0  SampleTime=0.02
  Selector1 : Selector  InputPortWidth=4  IndexOptions=Index vector (dialog)  Indices=[4]  OutputSizes=1
  Selector2 : Selector  InputPortWidth=4  IndexOptions=Index vector (dialog)  Indices=[1 2 3]  OutputSizes=1
  Selector3 : Selector  InputPortWidth=4  IndexOptions=Index vector (dialog)  Indices=[1 2 3]  OutputSizes=1
  Square(omega) : Gain  Gain=Omega_r^2
  Sum : Sum  Inputs=|+-
  Sum1 : Sum  Inputs=|+-
  acc lim : Saturate  UpperLimit=4  LowerLimit=-4
  position des : Outport
  attitude des : Outport  Port=2
  velocity des : Outport  Port=3
  acc des : Outport  Port=4
  wires:
  Selector3/1 -> velocity des/1
  Mux/1 -> attitude des/1
  Selector1/1 -> Mux/3
  Pitch/1 -> Mux/2
  Roll/1 -> Mux/1
  Selector2/1 -> position des/1
  2*zeta*omega/1 -> Sum1/2
  Sum1/1 -> acc lim/1
  Discrete-Time Integrator/1 -> Discrete-Time Integrator1/1, Selector3/1, 2*zeta*omega/1
  Square(omega)/1 -> Sum1/1
  Sum/1 -> Square(omega)/1
  PosCom/1 -> Sum/1
  Discrete-Time Integrator1/1 -> Selector1/1, Selector2/1, Sum/2  "ComRef"
  acc lim/1 -> Discrete-Time Integrator/1, acc des/1

== system Demo_Multiple_Quad/Quad 4 Planning/Vertical Controller/Verticall Pos Controller ==
  note: 0.15
      | 0.08
      | 0.15
  note: Set 1:
      | with KF
  note: 0.25
      | 0.1
      | 0.15
  note: Set 1:
      | without KF
  Pos Error : Inport
  Reset : Inport  Port=2
  Vel Error : Inport  Port=3
  Hover Throttle : Inport  Port=4
  D Gain : Gain  Gain=0.1  OutDataTypeStr=double
  Integral Gain : Gain  DisableCoverage=on  Gain=0.05  ParamDataTypeStr=double  OutDataTypeStr=double
  Integrator : DiscreteIntegrator  DisableCoverage=on  IntegratorMethod=Integration: Trapezoidal  ExternalReset=rising  InitialConditionMode=State only (most efficient)  SampleTime=-1  OutDataTypeStr=double  LimitOutput=on  UpperSaturationLimit=0.3  LowerSaturationLimit=-0.3  ICPrevOutput=DiscIntNeverNeededParam  ICPrevScaledInput=DiscIntNeverNeededParam
  Proportional Gain : Gain  DisableCoverage=on  Gain=0.1  ParamDataTypeStr=double  OutDataTypeStr=double
  Sum1 : Sum  DisableCoverage=on  Inputs=---|  AccumDataTypeStr=double  OutDataTypeStr=double  SampleTime=0.02
  Sum2 : Sum  DisableCoverage=on  Inputs=++|  AccumDataTypeStr=double  OutDataTypeStr=double  SampleTime=0.02
  "T  Commands [0, 1]" : Outport
  wires:
  Sum2/1 -> "T  Commands [0, 1]"/1
  Hover Throttle/1 -> Sum2/2
  Sum1/1 -> Sum2/1
  D Gain/1 -> Sum1/3
  Vel Error/1 -> D Gain/1
  Reset/1 -> Integrator/2
  Pos Error/1 -> Integral Gain/1, Proportional Gain/1
  Proportional Gain/1 -> Sum1/1
  Integrator/1 -> Sum1/2
  Integral Gain/1 -> Integrator/1

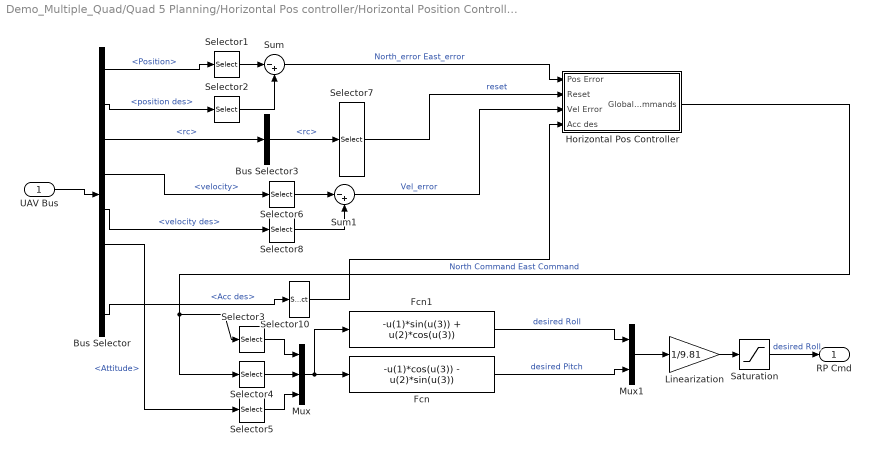
== system Demo_Multiple_Quad/Quad 5 Planning/Horizontal Pos controller/Horizontal Position Controller ==
  UAV Bus : Inport
  Bus Selector : BusSelector  OutputSignals=Position,position des,rc,velocity,velocity des,Attitude,Acceleration,Acc des
  Bus Selector3 : BusSelector  OutputSignals=rc
  Fcn : Fcn  Expr=-u(1)*cos(u(3)) - u(2)*sin(u(3))
  Fcn1 : Fcn  Expr=-u(1)*sin(u(3)) + u(2)*cos(u(3))
  Horizontal Pos Controller : Subsystem
  Linearization : Gain  Gain=1/9.81  OutDataTypeStr=double
  Mux : Mux  Inputs=3
  Mux1 : Mux  Inputs=2
  Saturation : Saturate  UpperLimit=60*pi/180  LowerLimit=-60*pi/180
  Selector{1..2,6,8} (4 alike) : Selector  InputPortWidth=3  IndexOptions=Index vector (dialog)  Indices=[1 2]  OutputSizes=1
  Selector10 : Selector  InputPortWidth=4  IndexOptions=Index vector (dialog)  Indices=[1 2]  OutputSizes=1
  Selector3 : Selector  InputPortWidth=2  IndexOptions=Index vector (dialog)  Indices=[1]  OutputSizes=1
  Selector4 : Selector  InputPortWidth=2  IndexOptions=Index vector (dialog)  Indices=[2]  OutputSizes=1
  Selector5 : Selector  InputPortWidth=3  IndexOptions=Index vector (dialog)  Indices=[3]  OutputSizes=1
  Selector7 : Selector  InputPortWidth=8  IndexOptions=Index vector (dialog)  Indices=[7]  OutputSizes=1
  Sum : Sum  Inputs=|-+
  Sum1 : Sum  Inputs=|-+
  RP Cmd : Outport
  wires:
  Saturation/1 -> RP Cmd/1  "desired Roll"
  Linearization/1 -> Saturation/1
  Selector10/1 -> Horizontal Pos Controller/4(Acc des)
  Bus Selector/8 -> Selector10/1  "<Acc des>"
  Bus Selector/5 -> Selector8/1  "<velocity des>"
  Bus Selector/4 -> Selector6/1  "<velocity>"
  Bus Selector/3 -> Bus Selector3/1  "<rc>"
  Selector8/1 -> Sum1/2
  Selector6/1 -> Sum1/1
  Sum1/1 -> Horizontal Pos Controller/3(Vel Error)  "Vel_error"
  Selector7/1 -> Horizontal Pos Controller/2(Reset)  "reset"
  Bus Selector3/1 -> Selector7/1  "<rc>"
  Mux1/1 -> Linearization/1
  Fcn/1 -> Mux1/2  "desired Pitch"
  Fcn1/1 -> Mux1/1  "desired Roll"
  Mux/1 -> Fcn1/1, Fcn/1
  Selector5/1 -> Mux/3
  Selector4/1 -> Mux/2
  Selector3/1 -> Mux/1
  Bus Selector/6 -> Selector5/1  "<Attitude>"
  Horizontal Pos Controller/1(Global Commands) -> Selector4/1, Selector3/1  "North Command East Command"
  UAV Bus/1 -> Bus Selector/1
  Selector2/1 -> Sum/2
  Selector1/1 -> Sum/1
  Bus Selector/2 -> Selector2/1  "<position des>"
  Bus Selector/1 -> Selector1/1  "<Position>"
  Sum/1 -> Horizontal Pos Controller/1(Pos Error)  "North_error East_error"

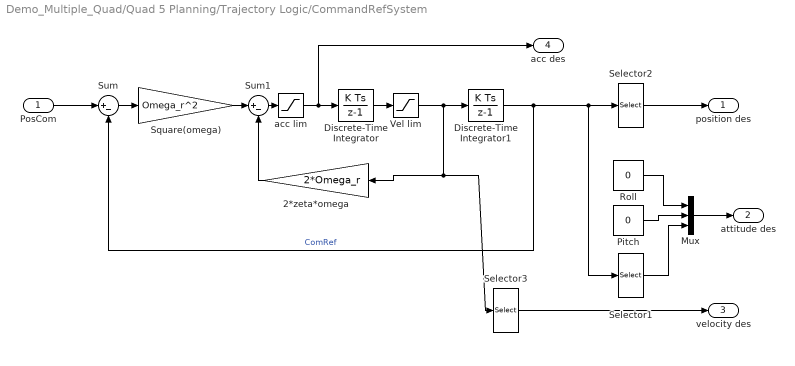
== system Demo_Multiple_Quad/Quad 5 Planning/Trajectory Logic/CommandRefSystem ==
  PosCom : Inport
  2*zeta*omega : Gain  Gain=2*Omega_r
  Discrete-Time Integrator : DiscreteIntegrator  SampleTime=0.02  ICPrevOutput=DiscIntNeverNeededParam  ICPrevScaledInput=DiscIntNeverNeededParam
  Discrete-Time Integrator1 : DiscreteIntegrator  SampleTime=0.02  ICPrevOutput=DiscIntNeverNeededParam  ICPrevScaledInput=DiscIntNeverNeededParam
  Mux : Mux  Inputs=3
  Pitch : Constant  Value=0  SampleTime=0.02
  Roll : Constant  Value=0  SampleTime=0.02
  Selector1 : Selector  InputPortWidth=4  IndexOptions=Index vector (dialog)  Indices=[4]  OutputSizes=1
  Selector2 : Selector  InputPortWidth=4  IndexOptions=Index vector (dialog)  Indices=[1 2 3]  OutputSizes=1
  Selector3 : Selector  InputPortWidth=4  IndexOptions=Index vector (dialog)  Indices=[1 2 3]  OutputSizes=1
  Square(omega) : Gain  Gain=Omega_r^2
  Sum : Sum  Inputs=|+-
  Sum1 : Sum  Inputs=|+-
  Vel lim : Saturate  UpperLimit=3  LowerLimit=-3
  acc lim : Saturate  UpperLimit=4  LowerLimit=-4
  position des : Outport
  attitude des : Outport  Port=2
  velocity des : Outport  Port=3
  acc des : Outport  Port=4
  wires:
  Vel lim/1 -> Discrete-Time Integrator1/1, Selector3/1, 2*zeta*omega/1
  acc lim/1 -> Discrete-Time Integrator/1, acc des/1
  Selector3/1 -> velocity des/1
  Mux/1 -> attitude des/1
  Selector1/1 -> Mux/3
  Pitch/1 -> Mux/2
  Roll/1 -> Mux/1
  Selector2/1 -> position des/1
  2*zeta*omega/1 -> Sum1/2
  Sum1/1 -> acc lim/1
  Discrete-Time Integrator/1 -> Vel lim/1
  Square(omega)/1 -> Sum1/1
  Sum/1 -> Square(omega)/1
  PosCom/1 -> Sum/1
  Discrete-Time Integrator1/1 -> Selector1/1, Selector2/1, Sum/2  "ComRef"

== system Demo_Multiple_Quad/Quad 5 Planning/Vertical Controller/Verticall Pos Controller ==
  note: 0.15
      | 0.08
      | 0.15
  note: Set 1:
      | with KF
  note: 0.25
      | 0.1
      | 0.15
  note: Set 1:
      | without KF
  Pos Error : Inport
  Reset : Inport  Port=2
  Vel Error : Inport  Port=3
  Hover Throttle : Inport  Port=4
  D Gain : Gain  Gain=0.1  OutDataTypeStr=double
  Integral Gain : Gain  DisableCoverage=on  Gain=0.05  ParamDataTypeStr=double  OutDataTypeStr=double
  Integrator : DiscreteIntegrator  DisableCoverage=on  IntegratorMethod=Integration: Trapezoidal  ExternalReset=rising  InitialConditionMode=State only (most efficient)  SampleTime=-1  OutDataTypeStr=double  LimitOutput=on  UpperSaturationLimit=0.3  LowerSaturationLimit=-0.3  ICPrevOutput=DiscIntNeverNeededParam  ICPrevScaledInput=DiscIntNeverNeededParam
  Proportional Gain : Gain  DisableCoverage=on  Gain=0.1  ParamDataTypeStr=double  OutDataTypeStr=double
  Sum1 : Sum  DisableCoverage=on  Inputs=---|  AccumDataTypeStr=double  OutDataTypeStr=double  SampleTime=0.02
  Sum2 : Sum  DisableCoverage=on  Inputs=++|  AccumDataTypeStr=double  OutDataTypeStr=double  SampleTime=0.02
  "T  Commands [0, 1]" : Outport
  wires:
  Sum2/1 -> "T  Commands [0, 1]"/1
  Hover Throttle/1 -> Sum2/2
  Sum1/1 -> Sum2/1
  D Gain/1 -> Sum1/3
  Vel Error/1 -> D Gain/1
  Reset/1 -> Integrator/2
  Pos Error/1 -> Integral Gain/1, Proportional Gain/1
  Proportional Gain/1 -> Sum1/1
  Integrator/1 -> Sum1/2
  Integral Gain/1 -> Integrator/1

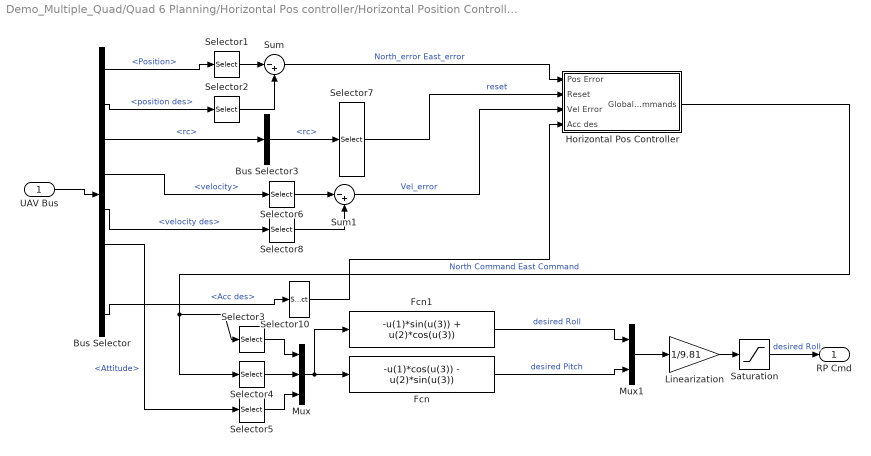
== system Demo_Multiple_Quad/Quad 6 Planning/Horizontal Pos controller/Horizontal Position Controller ==
  UAV Bus : Inport
  Bus Selector : BusSelector  OutputSignals=Position,position des,rc,velocity,velocity des,Attitude,Acceleration,Acc des
  Bus Selector3 : BusSelector  OutputSignals=rc
  Fcn : Fcn  Expr=-u(1)*cos(u(3)) - u(2)*sin(u(3))
  Fcn1 : Fcn  Expr=-u(1)*sin(u(3)) + u(2)*cos(u(3))
  Horizontal Pos Controller : Subsystem
  Linearization : Gain  Gain=1/9.81  OutDataTypeStr=double
  Mux : Mux  Inputs=3
  Mux1 : Mux  Inputs=2
  Saturation : Saturate  UpperLimit=60*pi/180  LowerLimit=-60*pi/180
  Selector{1..2,6,8} (4 alike) : Selector  InputPortWidth=3  IndexOptions=Index vector (dialog)  Indices=[1 2]  OutputSizes=1
  Selector10 : Selector  InputPortWidth=4  IndexOptions=Index vector (dialog)  Indices=[1 2]  OutputSizes=1
  Selector3 : Selector  InputPortWidth=2  IndexOptions=Index vector (dialog)  Indices=[1]  OutputSizes=1
  Selector4 : Selector  InputPortWidth=2  IndexOptions=Index vector (dialog)  Indices=[2]  OutputSizes=1
  Selector5 : Selector  InputPortWidth=3  IndexOptions=Index vector (dialog)  Indices=[3]  OutputSizes=1
  Selector7 : Selector  InputPortWidth=8  IndexOptions=Index vector (dialog)  Indices=[7]  OutputSizes=1
  Sum : Sum  Inputs=|-+
  Sum1 : Sum  Inputs=|-+
  RP Cmd : Outport
  wires:
  Saturation/1 -> RP Cmd/1  "desired Roll"
  Linearization/1 -> Saturation/1
  Selector10/1 -> Horizontal Pos Controller/4(Acc des)
  Bus Selector/8 -> Selector10/1  "<Acc des>"
  Bus Selector/5 -> Selector8/1  "<velocity des>"
  Bus Selector/4 -> Selector6/1  "<velocity>"
  Bus Selector/3 -> Bus Selector3/1  "<rc>"
  Selector8/1 -> Sum1/2
  Selector6/1 -> Sum1/1
  Sum1/1 -> Horizontal Pos Controller/3(Vel Error)  "Vel_error"
  Selector7/1 -> Horizontal Pos Controller/2(Reset)  "reset"
  Bus Selector3/1 -> Selector7/1  "<rc>"
  Mux1/1 -> Linearization/1
  Fcn/1 -> Mux1/2  "desired Pitch"
  Fcn1/1 -> Mux1/1  "desired Roll"
  Mux/1 -> Fcn1/1, Fcn/1
  Selector5/1 -> Mux/3
  Selector4/1 -> Mux/2
  Selector3/1 -> Mux/1
  Bus Selector/6 -> Selector5/1  "<Attitude>"
  Horizontal Pos Controller/1(Global Commands) -> Selector4/1, Selector3/1  "North Command East Command"
  UAV Bus/1 -> Bus Selector/1
  Selector2/1 -> Sum/2
  Selector1/1 -> Sum/1
  Bus Selector/2 -> Selector2/1  "<position des>"
  Bus Selector/1 -> Selector1/1  "<Position>"
  Sum/1 -> Horizontal Pos Controller/1(Pos Error)  "North_error East_error"
